simulink model "AM_SSB_SC_DEMODULATION"  (R2024a)
settings: Solver=VariableStepAuto  StartTime=0.0  StopTime=10.0  RelTol=1e-3
libraries: dspfdesign x1
settings Model: Creator=zeyad  LastModifiedBy=zeyad

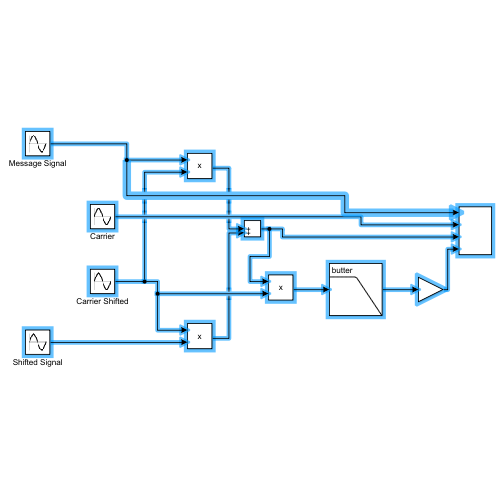
[thumbnail: Simulink's stored preview of the top-level diagram]
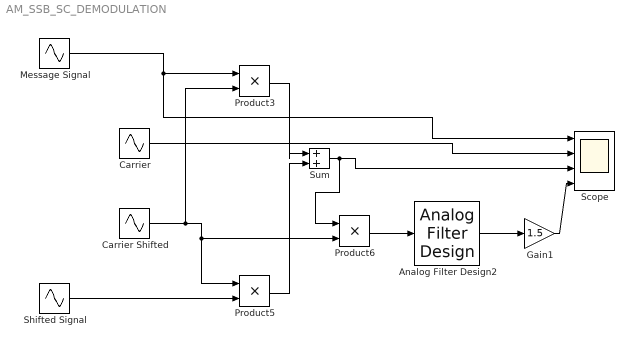
== system AM_SSB_SC_DEMODULATION ==
  Analog Filter Design2 : dspfdesign/Analog Filter Design  method=Butterworth  filttype=Lowpass  N=8  Wlo=60  Whi=80  Rp=2  Rs=40
  Carrier : Sin  Frequency=100  SampleTime=0
  Carrier Shifted : Sin  Frequency=100  Phase=-(pi/2)  SampleTime=0
  Gain1 : Gain  Gain=1.5
  Message Signal : Sin  Frequency=5  SampleTime=0
  Product3 : Product
  Product5 : Product
  Product6 : Product
  Scope : Scope  NumInputPorts=4
  Shifted Signal : Sin  Frequency=5  Phase=-(pi/2)  SampleTime=0
  Sum : Sum  Inputs=|++
  wires:
  Gain1/1 -> Scope/4
  Analog Filter Design2/1 -> Gain1/1
  Sum/1 -> Product6/1, Scope/3
  Carrier Shifted/1 -> Product3/2, Product6/2, Product5/1
  Product5/1 -> Sum/2
  Shifted Signal/1 -> Product5/2
  Carrier/1 -> Scope/2
  Product3/1 -> Sum/1
  Product6/1 -> Analog Filter Design2/1
  Message Signal/1 -> Scope/1, Product3/1
